simulink model "RollAutopilotRevised"  (R2017a)
settings: Solver=FixedStepDiscrete  StartTime=0.0  StopTime=25  FixedStep=1/40  RelTol=1e-3
PreLoadFcn:
  | load RollRefInputAP.mat
  | load RollRefInputPhi.mat
  | load RollRefInputTK.mat
model workspace (MAT data in the model file):
  dispGain = Simulink.Parameter
  dispGain.Value = 1
  dispGain.DataType = 'auto'
  dispGain.Dimensions = [1 1]
  hdgGain = Simulink.Parameter
  hdgGain.Value = 0.015
  hdgGain.DataType = 'auto'
  hdgGain.Min = 0
  hdgGain.Dimensions = [1 1]
  intGain = Simulink.Parameter
  intGain.Value = 1
  intGain.DataType = 'auto'
  intGain.Dimensions = [1 1]
  rateGain = Simulink.Parameter
  rateGain.Value = 3
  rateGain.DataType = 'auto'
  rateGain.Dimensions = [1 1]
undefined symbols (not defined in the file or in its folder): cmdLim, dispLim, intLim, rateLim
libraries: simulink x1, simulink_need_slupdate x1
settings Model: RequirementInfo={} %GIDa_fe9045fd_0412_4b6e_8206_617cc20e6fde  ParameterArgumentNames=dispGain,intGain,rateGain,hdgGain  Creator=The MathWorks, Inc.  LastModifiedBy=The MathWorks, Inc.
settings DataIOCC: ExternalInput=rollIn  SaveFormat=StructureWithTime  SaveOutput=off  DSMLogging=off  ReturnWorkspaceOutputs=on  OutputSaveName=Ail_Cmd  SignalLoggingName=sltlogsout
settings OptimizationCC: BlockReduction=off  DefaultParameterBehavior=Inlined  InlineInvariantSignals=on  ExpressionDepthLimit=2147483647  EfficientFloat2IntCast=on  EfficientMapNaN2IntZero=off  LifeSpan=inf  MaxStackSize=inf
settings DebuggingCC: SignalInfNanChecking=error  SignalRangeChecking=error  ReadBeforeWriteMsg=EnableAllAsError  WriteAfterWriteMsg=EnableAllAsError  WriteAfterReadMsg=EnableAllAsError  AlgebraicLoopMsg=error  ArtificialAlgebraicLoopMsg=error  SaveWithDisabledLinksMsg=error  SaveWithParameterizedLinksMsg=error  CheckExecutionContextPreStartOutputMsg=on  CheckExecutionContextRuntimeOutputMsg=on  BlockPriorityViolationMsg=error  MaxConsecutiveZCsMsg=warning  SolverPrmCheckMsg=error  InheritedTsInSrcMsg=error  SingleTaskRateTransMsg=error  TasksWithSamePriorityMsg=error  SigSpecEnsureSampleTimeMsg=error  CheckMatrixSingularityMsg=error  IntegerOverflowMsg=error  ParameterUnderflowMsg=error  ParameterPrecisionLossMsg=error  ParameterTunabilityLossMsg=error  UnderSpecifiedDataTypeMsg=error  UnnecessaryDatatypeConvMsg=warning  VectorMatrixConversionMsg=error  SignalLabelMismatchMsg=error  UnconnectedInputMsg=error  UnconnectedOutputMsg=error  UnconnectedLineMsg=error  SFcnCompatibilityMsg=error  UniqueDataStoreMsg=error  BusObjectLabelMismatch=error  RootOutportRequireBusObject=error  AssertControl=DisableAll  AllowSymbolicDim=off  ModelReferenceIOMsg=error  ModelReferenceIOMismatchMessage=error  UnknownTsInhSupMsg=error  ModelReferenceDataLoggingMessage=error  ModelReferenceExtraNoncontSigs=none  StateNameClashWarn=warning  StrictBusMsg=ErrorOnBusTreatedAsVector  NonBusSignalsTreatedAsBus=error  SFUnexpectedBacktrackingDiag=warning  SFNoUnconditionalDefaultTransitionDiag=warning  SFExecutionAtInitializationDiag=none  IntegerSaturationMsg=error
settings HardwareCC: ProdBitPerPointer=32  ProdLargestAtomicFloat=None  ProdEndianess=BigEndian  ProdWordSize=32  ProdHWDeviceType=32-bit Embedded Processor  TargetHWDeviceType=32-bit Generic
settings ModelReferenceCC: PropagateSignalLabelsOutOfModel=off
settings SFSimCC: MATLABDynamicMemAlloc=off
settings RTWCC: SystemTargetFile=ert.tlc  TemplateMakefile=ert_default_tmf  Description=Embedded Coder  GenerateReport=on  RTWVerbose=off  IncludeHyperlinkInReport=on  LaunchReport=on  PortableWordSizes=on  GenerateTraceInfo=on  GenerateTraceReport=on  GenerateTraceReportSl=on  GenerateTraceReportSf=on  GenerateTraceReportEml=on
settings CodeAppCC: ForceParamTrailComments=on  IgnoreCustomStorageClasses=off  MaxIdLength=63  MangleLength=4  CustomSymbolStrType=$N$R$M  InternalIdentifier=Classic  ReqsInCode=on
settings ERTTargetCC: UtilityFuncGeneration=Shared location  MultiwordLength=2048  IncludeMdlTerminateFcn=off  GeneratePreprocessorConditionals=Disable all  SuppressErrorStatus=on  SupportAbsoluteTime=off  SupportNonFinite=off  SupportComplex=off  ParenthesesLevel=Maximum  MultiInstanceErrorCode=None  ERTCustomFileTemplate=example_file_process.tlc  PreserveExpressionOrder=on  PreserveIfCondition=on  ConvertIfToSwitch=off  SuppressUnreachableDefaultCases=off
settings ConfigComp: CovEnable=on  CovScope=Subsystem  RecordCoverage=on  CovPath=Roll Reference  CovSaveName=covdata_rollAP  CovMetricSettings=dcwe  CovHTMLOptions=-sRT=0 -sVT=0 -aTS=1 -bRG=1 -bTC=1 -hTR=1 -nFC=0 -nFD=1 -scm=1 -bcm=1 -xEv=0 -xEM=0  CovHtmlReporting=on  CovSaveCumulativeToWorkspaceVar=on  CovSaveSingleToWorkspaceVar=on  CovCumulativeVarName=covCumulativeData_rollAP  CovCumulativeReport=on  CovReportOnPause=off  CovExternalEMLEnable=off  CovSFcnEnable=off  PSOpenProjectManager=on  PSSendToPolyspaceServer=on  PSModelRefVerifDepth=All  PSAutoStubLUT=off  DVMakeOutputFilesUnique=off  DVModelCoverageObjectives=None  DVMaxTestCaseSteps=500  DVTestSuiteOptimization=CombinedObjectives (Nonlinear Extended)  DVCoverageDataFile=existingcov.cvt  DVIncludeRelationalBoundary=on  DVDetectFloatOverflow=off  DVSaveDataFile=off  DVModelReferenceHarness=on  DVSaveReport=on  DVSFcnSupport=off

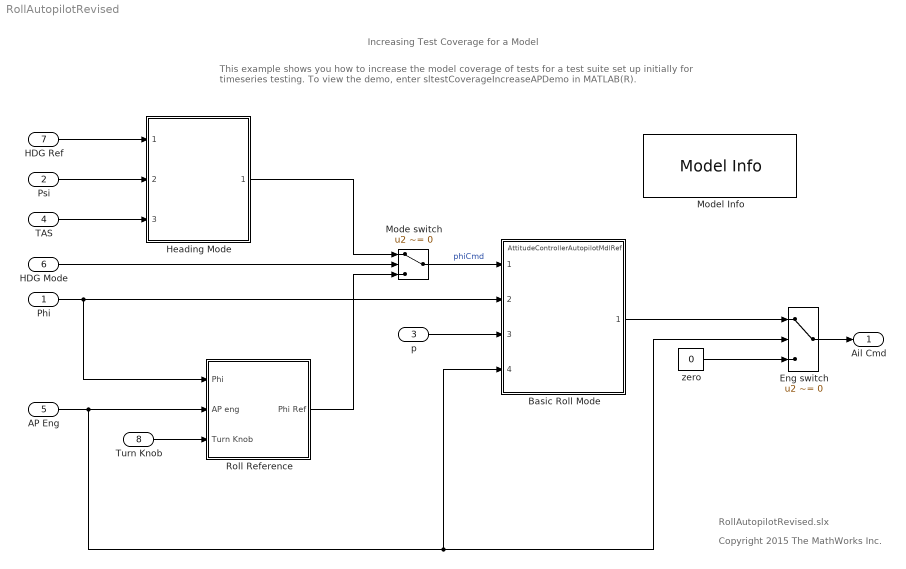
== system RollAutopilotRevised ==
  note: Copyright 2015 The MathWorks Inc.
  note: RollAutopilotRevised.slx
  note: This example shows you how to increase the model coverage of tests for a test suite set up initially for timeseries testing.
      | To view the demo, enter sltestCoverageIncreaseAPDemo in MATLAB(R).
  note: Increasing Test Coverage for a Model
  Phi : Inport  RequirementInfo={'other' 'do178b_autopilot_requirements.docx' '@Simulink_requirement_item_3' 'true' '1.3. Roll Hold Reference' ' ' ; 'other' 'do178b_autopilot_requirements.docx' '@Simulink_requirement_item_4' 'true' '1.4. Roll Performance' '' } %GIDa_040c2d73_6311_42f9_964f_56f1fff3d8d8  OutMin=-180  OutMax=180  OutDataTypeStr=double  PortDimensions=1  SampleTime=1/40  Interpolate=off
  Psi : Inport  RequirementInfo={'other' 'do178b_autopilot_requirements.docx' '@Simulink_requirement_item_10' 'true' '1.10. Heading Performance' '' } %GIDa_aa699f91_96f0_401b_acdb_f9b4b0743533  Port=2  OutMin=-180  OutMax=180  OutDataTypeStr=double  PortDimensions=1  SampleTime=1/40  Interpolate=off
  p : Inport  RequirementInfo={'other' 'do178b_autopilot_requirements.docx' '@Simulink_requirement_item_4' 'true' '1.4. Roll Performance' '' } %GIDa_91b6e343_cedd_4c09_9e82_9cc09e4312a7  Port=3  OutMin=-180  OutMax=180  OutDataTypeStr=double  PortDimensions=1  SampleTime=1/40  Interpolate=off
  TAS : Inport  RequirementInfo={'other' 'do178b_autopilot_requirements.docx' '@Simulink_requirement_item_10' 'true' '1.10. Heading Performance' '' } %GIDa_9daa2c3d_09c1_4ac6_a206_1425f5f778cd  Port=4  OutMin=0  OutMax=1000  OutDataTypeStr=double  PortDimensions=1  SampleTime=1/40  Interpolate=off
  AP Eng : Inport  RequirementInfo={'other' 'do178b_autopilot_requirements.docx' '@Simulink_requirement_item_1' 'true' '1.1. Roll Autopilot Engage Control' ' ' ; 'other' 'do178b_autopilot_requirements.docx' '@Simulink_requirement_item_3' 'true' '1.3. Roll Hold Reference' ' ' ; 'other' 'do178b_autopilot_requirements.docx' '@Simulink_requirement_item_4' 'true' '1.4. Roll Performance' '' } %GIDa_dbf8c750_871c_42fc_8ea1_57838e97fa97  Port=5  OutDataTypeStr=boolean  PortDimensions=1  SampleTime=1/40  Interpolate=off
  HDG Mode : Inport  RequirementInfo={'other' 'do178b_autopilot_requirements.docx' '@Simulink_requirement_item_2' 'true' '1.2. Roll Hold Mode' ' ' ; 'other' 'do178b_autopilot_requirements.docx' '@Simulink_requirement_item_8' 'true' '1.8. Heading Hold Mode' '' } %GIDa_3d1fd2be_b046_42ef_8f3c_1955bceadbb7  Port=6  OutDataTypeStr=boolean  PortDimensions=1  SampleTime=1/40  Interpolate=off
  HDG Ref : Inport  RequirementInfo={'other' 'do178b_autopilot_requirements.docx' '@Simulink_requirement_item_9' 'true' '1.9. Heading Hold Reference' ' ' ; 'other' 'do178b_autopilot_requirements.docx' '@Simulink_requirement_item_10' 'true' '1.10. Heading Performance' '' } %GIDa_96162cda_cb1a_490e_8dac_f861526aad50  Port=7  OutMin=-180  OutMax=180  OutDataTypeStr=double  PortDimensions=1  SampleTime=1/40  Interpolate=off
  Turn Knob : Inport  RequirementInfo={'other' 'do178b_autopilot_requirements.docx' '@Simulink_requirement_item_3' 'true' '1.3. Roll Hold Reference' '' } %GIDa_fa976ccd_1ea9_4823_b673_fef2768ad601  Port=8  OutMin=-45  OutMax=45  OutDataTypeStr=double  PortDimensions=1  SampleTime=1/40  Interpolate=off
  Basic Roll Mode : ModelReference  RequirementInfo={'other' 'do178b_autopilot_requirements.docx' '@Simulink_requirement_item_4' 'true' '1.4. Roll Performance' '' ; 'other' 'do178b_autopilot_requirements.docx' '@Simulink_requirement_item_5' 'true' '1.5. Roll Rate Limit' '' ; 'other' 'do178b_autopilot_requirements.docx' '@Simulink_requirement_item_6' 'true' '1.6. Roll Angle Limit' '' ; 'other' 'do178b_autopilot_requirements.docx' '@Simulink_requirement_item_7' 'true' '1.7. Aileron Angle Limit' '' } %GIDa_94fed7b0_f432_43f5_a2d9_2abccf075f5b  ModelNameDialog=AttitudeControllerAutopilotMdlRef.slx  ParameterArgumentNames=cmdLim,dispGain,dispLim,intGain,intLim,rateGain,rateLim  ParameterArgumentValues=15,dispGain,30,intGain,5,rateGain,6  UsingDefaultArgumentValue=0,0,0,0,0,0,0  SimulationMode=Normal  ModelReferenceVersion=1.73
  Eng switch : Switch  RequirementInfo={'other' 'do178b_autopilot_requirements.docx' '' 'true' '1.1. Roll Autopilot Engage Control' ' ' } %GIDa_1f89e2a1_f10b_411b_80f1_4c7070559f04  Criteria=u2 ~= 0
  Heading Mode : ModelReference  RequirementInfo={'other' 'do178b_autopilot_requirements.docx' '@Simulink_requirement_item_10' 'true' '1.10. Heading Performance' '' } %GIDa_e0954c89_e814_46d2_8f67_6d4b1cdfab81  ModelNameDialog=HeadingModeAutopilotMdlRef.slx  ParameterArgumentNames=hdgGain  ParameterArgumentValues=hdgGain  UsingDefaultArgumentValue=0  SimulationMode=Normal  ModelReferenceVersion=1.152
  Mode switch : Switch  RequirementInfo={'other' 'do178b_autopilot_requirements.docx' '@Simulink_requirement_item_2' 'true' '1.2. Roll Hold Mode' ' ' ; 'other' 'do178b_autopilot_requirements.docx' '@Simulink_requirement_item_4' 'true' '1.4. Roll Performance' ' ' ; 'other' 'do178b_autopilot_requirements.docx' '@Simulink_requirement_item_8' 'true' '1.8. Heading Hold Mode' ' ' ; 'other' 'do178b_autopilot_requirements.docx' '@Simulink_requirement_item_10' 'true' '1.10. Heading Performance' '' } %GIDa_89518de0_411a_4ee8_869d_c7ed5e5087e3  Criteria=u2 ~= 0
  Model Info : simulink/Model-Wide Utilities/Model Info  RequirementInfo={} %GIDa_ca11a4b2_f22f_461f_8532_eb2c7aa53101  InitialSaveTempField=(Not available in SLX model file format)#|#(Not available in SLX model file format)#|#(Not available in SLX model file format)#|#(Not available in SLX model file format)#|#(Not available in SLX model file format)#|#(Not available in SLX model file format)#|#(Not available in SLX model file format)#|#(Not available in SLX model file format)#|#(Not available in SLX model file format)#|#  InitialBlockCM=Microsoft Visual SourceSafe  BlockCM=Microsoft Visual SourceSafe  Frame=on  SaveTempField=(Not available in SLX model file format)#|#(Not available in SLX model file format)#|#(Not available in SLX model file format)#|#(Not available in SLX model file format)#|#(Not available in SLX model file format)#|#(Not available in SLX model file format)#|#(Not available in SLX model file format)#|#(Not available in SLX model file format)#|#(Not available in SLX model file format)#|#  DisplayStringWithTags=|  HorizontalTextAlignment=Left  LeftAlignmentValue=0.02  SourceBlockDiagram=RollAutopilotRevised  TagMaxNumber=20  CMTag1=$Author: $  CMTag2=$Date: $  CMTag3=$Revision: $  CMTag4=$Archive: $  CMTag5=$Header: $  CMTag6=$Logfile: $  CMTag7=$Modtime: $  CMTag8=$Workfile: $  CMTag9=$JustDate: $
      | Roll Autopilot Revised
      | Author: %<LastModifiedBy>
      | Model Version: %<ModelVersion>
      | Date: %<LastModificationDate>
  Roll Reference : Subsystem  RequirementInfo={'other' 'do178b_autopilot_requirements.docx' '@Simulink_requirement_item_3' 'true' '1.3. Roll Hold Reference' '' } %GIDa_c8cf196e_df7c_4434_8b0c_5575b514a7cf  TreatAsAtomicUnit=on
      settings: RTWSystemCode=Inline
  zero : Constant  RequirementInfo={'other' 'do178b_autopilot_requirements.docx' '' 'true' '1.1. Roll Autopilot Engage Control' '' } %GIDa_8c99e557_6257_4659_beae_770a67a6ac3a  Value=0  OutDataTypeStr=double
  Ail Cmd : Outport  RequirementInfo={'other' 'do178b_autopilot_requirements.docx' '' 'true' '1.1. Roll Autopilot Engage Control' ' ' } %GIDa_02b61f6d_71d4_4b0d_89ac_bfbca808eb5f  OutDataTypeStr=double  PortDimensions=1  SampleTime=1/40
  wires:
  HDG Ref/1 -> Heading Mode/1
  Phi/1 -> Roll Reference/1(Phi), Basic Roll Mode/2
  p/1 -> Basic Roll Mode/3
  Psi/1 -> Heading Mode/2
  TAS/1 -> Heading Mode/3
  Mode switch/1 -> Basic Roll Mode/1  "phiCmd"
  HDG Mode/1 -> Mode switch/2
  Heading Mode/1 -> Mode switch/1
  AP Eng/1 -> Eng switch/2, Basic Roll Mode/4, Roll Reference/2(AP eng)
  Basic Roll Mode/1 -> Eng switch/1
  Eng switch/1 -> Ail Cmd/1
  zero/1 -> Eng switch/3
  Roll Reference/1(Phi Ref) -> Mode switch/3
  Turn Knob/1 -> Roll Reference/3(Turn Knob)

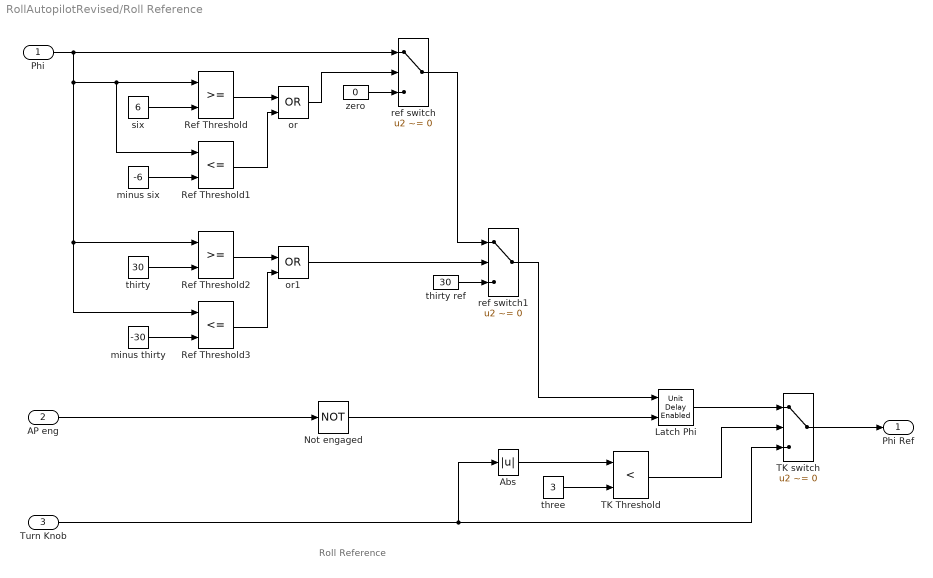
== system RollAutopilotRevised/Roll Reference ==
  note: Roll Reference
  Phi : Inport  RequirementInfo={'other' 'do178b_autopilot_requirements.docx' '@Simulink_requirement_item_3' 'true' '1.3. Roll Hold Reference' '' } %GIDa_365246ee_5fe4_4d20_a97b_c1028127f0f0
  AP eng : Inport  RequirementInfo={'other' 'do178b_autopilot_requirements.docx' '@Simulink_requirement_item_3' 'true' '1.3. Roll Hold Reference' '' } %GIDa_d4efac82_9df2_4cb3_8b82_71e18ecb0348  Port=2
  Turn Knob : Inport  RequirementInfo={'other' 'do178b_autopilot_requirements.docx' '@Simulink_requirement_item_3' 'true' '1.3. Roll Hold Reference' '' } %GIDa_d8bc0518_f9fa_4c47_a645_e8b5f2762f20  Port=3
  Abs : Abs  RequirementInfo={'other' 'do178b_autopilot_requirements.docx' '@Simulink_requirement_item_3' 'true' '1.3. Roll Hold Reference' '' } %GIDa_c8abfe5d_55a5_4c1b_9135_acd6c20e2232
  Latch Phi : simulink_need_slupdate/Unit Delay Enabled  RequirementInfo={'other' 'do178b_autopilot_requirements.docx' '@Simulink_requirement_item_3' 'true' '1.3. Roll Hold Reference' '' } %GIDa_8c2a6474_62f7_4673_9b80_815aaee792d7  vinit=0.0  tsamp=1/40
      settings: SourceProductName=Simulink  SourceProductBaseCode=SL
  Not engaged : Logic  RequirementInfo={'other' 'do178b_autopilot_requirements.docx' '@Simulink_requirement_item_3' 'true' '1.3. Roll Hold Reference' '' } %GIDa_e52c6893_d81b_4f15_89c3_12b6a83c27b2  Operator=NOT  IconShape=distinctive  AllPortsSameDT=off  OutDataTypeStr=boolean
  Ref Threshold : RelationalOperator  RequirementInfo={'other' 'do178b_autopilot_requirements.docx' '@Simulink_requirement_item_3' 'true' '1.3. Roll Hold Reference' '' } %GIDa_b5d668e1_6ee9_454f_ad19_deb7fa461421  OutDataTypeStr=boolean  RndMeth=Nearest  InputSameDT=on
  Ref Threshold1 : RelationalOperator  RequirementInfo={'other' 'do178b_autopilot_requirements.docx' '@Simulink_requirement_item_3' 'true' '1.3. Roll Hold Reference' '' } %GIDa_26a4d859_b01b_4f14_a8d9_5dd3bd1c8550  Operator=<=  OutDataTypeStr=boolean  RndMeth=Nearest  InputSameDT=on
  Ref Threshold2 : RelationalOperator  RequirementInfo={'other' 'do178b_autopilot_requirements.docx' '@Simulink_requirement_item_3' 'true' '1.3. Roll Hold Reference' '' } %GIDa_836e8f61_20f5_48a1_b010_9f972ca626b9  OutDataTypeStr=boolean  RndMeth=Nearest  InputSameDT=on
  Ref Threshold3 : RelationalOperator  RequirementInfo={'other' 'do178b_autopilot_requirements.docx' '@Simulink_requirement_item_3' 'true' '1.3. Roll Hold Reference' '' } %GIDa_c188cb95_81ce_47d3_b69e_464f67b2c913  Operator=<=  OutDataTypeStr=boolean  RndMeth=Nearest  InputSameDT=on
  TK Threshold : RelationalOperator  RequirementInfo={'other' 'do178b_autopilot_requirements.docx' '@Simulink_requirement_item_3' 'true' '1.3. Roll Hold Reference' '' } %GIDa_9859b478_272f_4974_a36c_6c4f8c030643  Operator=<  OutDataTypeStr=boolean  RndMeth=Nearest  InputSameDT=on
  TK switch : Switch  RequirementInfo={'other' 'do178b_autopilot_requirements.docx' '@Simulink_requirement_item_3' 'true' '1.3. Roll Hold Reference' '' } %GIDa_804165d0_89eb_4919_a8d1_f2310004f7d9  Criteria=u2 ~= 0
  minus six : Constant  RequirementInfo={'other' 'do178b_autopilot_requirements.docx' '@Simulink_requirement_item_3' 'true' '1.3. Roll Hold Reference' '' } %GIDa_6533fc10_b359_4ec9_aad4_622947196a15  Value=-6
  minus thirty : Constant  RequirementInfo={'other' 'do178b_autopilot_requirements.docx' '@Simulink_requirement_item_3' 'true' '1.3. Roll Hold Reference' '' } %GIDa_6f3ac5de_062d_4113_9269_f2542a8a139d  Value=-30
  or : Logic  RequirementInfo={'other' 'do178b_autopilot_requirements.docx' '@Simulink_requirement_item_3' 'true' '1.3. Roll Hold Reference' '' } %GIDa_f3b9166b_73be_49ce_a616_e5c65dca0ce4  Operator=OR  IconShape=distinctive  OutDataTypeStr=boolean
  or1 : Logic  RequirementInfo={'other' 'do178b_autopilot_requirements.docx' '@Simulink_requirement_item_3' 'true' '1.3. Roll Hold Reference' '' } %GIDa_1af6cde8_c206_4350_91a5_0c21c6d6c369  Operator=OR  IconShape=distinctive  OutDataTypeStr=boolean
  ref switch : Switch  RequirementInfo={'other' 'do178b_autopilot_requirements.docx' '@Simulink_requirement_item_3' 'true' '1.3. Roll Hold Reference' '' } %GIDa_a4746381_6ebe_4e3d_83b9_b49d14a3af5e  Criteria=u2 ~= 0
  ref switch1 : Switch  RequirementInfo={'other' 'do178b_autopilot_requirements.docx' '@Simulink_requirement_item_3' 'true' '1.3. Roll Hold Reference' '' } %GIDa_a4746381_6ebe_4e3d_83b9_b49d14a3af5e  Criteria=u2 ~= 0
  six : Constant  RequirementInfo={'other' 'do178b_autopilot_requirements.docx' '@Simulink_requirement_item_3' 'true' '1.3. Roll Hold Reference' '' } %GIDa_5e53f516_2e58_4597_b53a_6c713a53b7fc  Value=6
  thirty : Constant  RequirementInfo={'other' 'do178b_autopilot_requirements.docx' '@Simulink_requirement_item_3' 'true' '1.3. Roll Hold Reference' '' } %GIDa_95aab7f2_bb74_46fe_954d_5260cddff86b  Value=30
  thirty ref : Constant  RequirementInfo={'other' 'do178b_autopilot_requirements.docx' '@Simulink_requirement_item_3' 'true' '1.3. Roll Hold Reference' '' } %GIDa_e4775650_e5c7_4c74_aef4_71c144af3cbc  Value=30
  three : Constant  RequirementInfo={'other' 'do178b_autopilot_requirements.docx' '@Simulink_requirement_item_3' 'true' '1.3. Roll Hold Reference' '' } %GIDa_6228e2c4_8022_4eaf_90d6_7c47f19fb0a2  Value=3  OutDataTypeStr=double
  zero : Constant  RequirementInfo={'other' 'do178b_autopilot_requirements.docx' '@Simulink_requirement_item_3' 'true' '1.3. Roll Hold Reference' '' } %GIDa_e4775650_e5c7_4c74_aef4_71c144af3cbc  Value=0
  Phi Ref : Outport  RequirementInfo={'other' 'do178b_autopilot_requirements.docx' '@Simulink_requirement_item_3' 'true' '1.3. Roll Hold Reference' '' } %GIDa_75cfa841_d3b7_422f_bd46_8ed4a58fc723
  wires:
  ref switch1/1 -> Latch Phi/1
  thirty ref/1 -> ref switch1/3
  or1/1 -> ref switch1/2
  Not engaged/1 -> Latch Phi/2
  ref switch/1 -> ref switch1/1
  Latch Phi/1 -> TK switch/1
  TK Threshold/1 -> TK switch/2
  Turn Knob/1 -> TK switch/3, Abs/1
  three/1 -> TK Threshold/2
  Abs/1 -> TK Threshold/1
  AP eng/1 -> Not engaged/1
  TK switch/1 -> Phi Ref/1
  zero/1 -> ref switch/3
  six/1 -> Ref Threshold/2
  Ref Threshold/1 -> or/1
  Ref Threshold1/1 -> or/2
  minus six/1 -> Ref Threshold1/2
  or/1 -> ref switch/2
  Phi/1 -> ref switch/1, Ref Threshold/1, Ref Threshold1/1, Ref Threshold3/1, Ref Threshold2/1
  thirty/1 -> Ref Threshold2/2
  Ref Threshold2/1 -> or1/1
  Ref Threshold3/1 -> or1/2
  minus thirty/1 -> Ref Threshold3/2
